simulink model "MATE_SynchronousMachine"  (R2024b)
settings: Solver=FixedStepDiscrete  StartTime=0.0  StopTime=6  FixedStep=Ts  RelTol=1e-4  EnableMultiTasking=on
PostLoadFcn:
  | Ts=25e-6;offset=4;
InitFcn:
  | Ts=25e-6;offset=4;
undefined symbols (not defined in the file): DiscIntNeverNeededParam, MATE, Phase, Rsnu, Single
libraries: fl_lib x58, nesl_utility x43, ee_lib x13, simetran x5, simetranss x3, powerlib_extras x3, simulink_extras x2, simulink x2
(part 1 of 4)
settings Model: ARTEMISmethode_block_infos=$$__separator__$$  Creator=by2815  LastModifiedBy=CD8435
settings SolverCC: AlgebraicLoopSolver=TrustRegion
settings DataIOCC: SaveFormat=Structure  SignalLoggingSaveFormat=ModelDataLogs  SaveOutput=off  SignalLogging=off  SaveTime=off  ReturnWorkspaceOutputs=off  SignalLoggingName=sigsOut
settings OptimizationCC: ExpressionDepthLimit=2147483647  InitFltsAndDblsToZero=on  LifeSpan=inf
settings DebuggingCC: SaveWithParameterizedLinksMsg=none  UnderspecifiedInitializationDetection=Classic  MergeDetectMultiDrivingBlocksExec=none  SignalResolutionControl=TryResolveAllWithWarning  MultiTaskDSMMsg=warning  MultiTaskCondExecSysMsg=none  FcnCallInpInsideContextMsg=warning  AllowSymbolicDim=off  StateNameClashWarn=warning  NonBusSignalsTreatedAsBus=error  SFUnexpectedBacktrackingDiag=warning  SFNoUnconditionalDefaultTransitionDiag=warning  SFExecutionAtInitializationDiag=none  ArithmeticOperatorsInVariantConditions=warning
settings HardwareCC: ProdBitPerPointer=32  ProdBitPerSizeT=32  ProdBitPerPtrDiffT=32  ProdLargestAtomicFloat=None  ProdIntDivRoundTo=Undefined  ProdEndianess=Unspecified  ProdWordSize=32  ProdHWDeviceType=32-bit Generic  TargetUnknown=on
settings ModelReferenceCC: EnableRefExpFcnMdlSchedulingChecks=on  PropagateSignalLabelsOutOfModel=off
settings SFSimCC: SimUseLocalCustomCode=off  CustomCodeUndefinedFunction=UseInterfaceOnly
settings RTWCC: RTWUseLocalCustomCode=off  GPUComputeCapability=3.5
settings CodeAppCC: StateflowObjectComments=on
settings GRTTargetCC: TargetFcnLib=ansi_tfl_tmw.mat  TargetLangStandard=C89/C90 (ANSI)  CombineOutputUpdateFcns=off  GRTInterface=on
settings ConfigComp: CovMetricSettings=dw  CovSaveCumulativeToWorkspaceVar=on  CovSaveSingleToWorkspaceVar=on  CovExternalEMLEnable=off
settings SimscapeCC: SimscapeNormalizeSystem=off

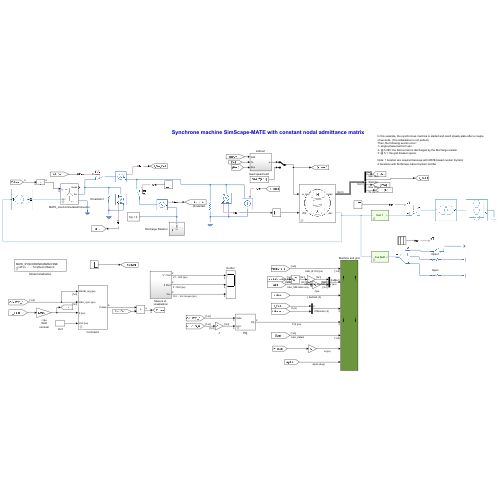
[thumbnail: Simulink's stored preview of the top-level diagram]
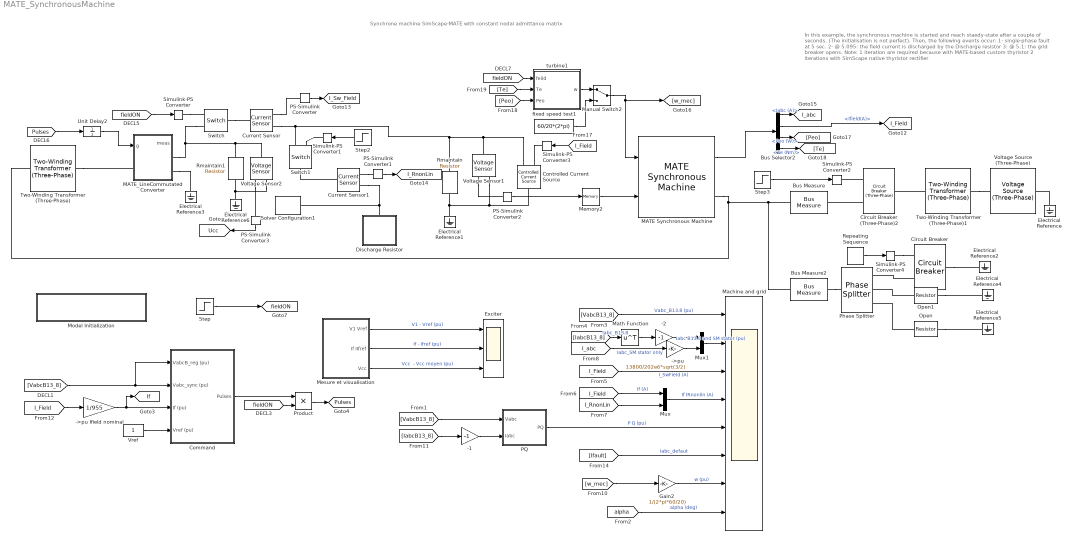
== system MATE_SynchronousMachine ==
  note: In this example, the synchronous machine is started and reach staedy-state after a couple of seconds. (The initialisation is not perfect).
      | Then, the following events occur:
      | 1- single-phase fault at 5 sec.
      | 2- @ 5.095: the field current is discharged by the Discharge resistor
      | 3: @ 5.1: the grid breaker opens.
      |
      | Note: 1 iteration are required because with MATE-based custom thyristor
      | 2 iterations with SimScape native thyristor rectifier
  note: Synchrone machine SimScape-MATE with constant nodal admittance matrix
  -1 : Gain  Gain=-1
  -2 : Gain  Gain=-1
  ->pu : Gain  Gain=13800/202e6*sqrt(3/2)
  ->pu Ifield nominal : Gain  Gain=1/955
  Bus Selector2 : BusSelector  OutputSignals=Iabc (A),Ifield(A),Peo (W),Te (Nm)
  Bus Measure : simetranss/Measure/Bus Measure  VoltageMeasurement=phase-to-ground  SetLabelV=on  LabelV=VabcB13_8  Vpu=on  VpuLL=off  CurrentMeasurement=yes  SetLabelI=on  LabelI=IabcB13_8  Ipu=on  Pbase=202e6  Vbase=13.8e3  bnumber=1  dis=off
  Bus Measure2 : simetranss/Measure/Bus Measure  VoltageMeasurement=phase-to-ground  SetLabelV=on  LabelV=Vfault  Vpu=off  VpuLL=off  CurrentMeasurement=yes  SetLabelI=on  LabelI=Ifault  Ipu=off  Pbase=202e6  Vbase=13.8e3  bnumber=fault  dis=off
  Circuit Breaker : ee_lib/Switches & Breakers/Circuit Breaker  R_closed=0.01 Ohm  G_open=1e-6 1/Ohm  threshold=0.5 V  breaker_behavior=ee.enum.switches.breakerBehavior.zeroCrossingEnable
      settings: InternalSimscapePortConfiguration="{\"Bottom\":[],\"Left\":[{\"id\":\"vT\",\"label\":\"vT\",\"type\":\"input\"},{\"id\":\"p1\",\"label\":\"\",\"type\":\"foundation.electrical.electrical\"}],\"Right\":[{\"id\":\"p2\",\"label\":\"\",\"type\":\"foundation.electrical.electrical\"}],\"Top\":[]}"
  Circuit Breaker (Three-Phase)2 : ee_lib/Switches & Breakers/Circuit Breaker (Three-Phase)  R_closed=0.01 Ohm  G_open=1e-6 1/Ohm  threshold=0.5 V  breaker_behavior=ee.enum.switches.breakerBehavior.zeroCrossingEnable
      settings: InternalSimscapePortConfiguration="{\"Bottom\":[],\"Left\":[{\"id\":\"vT\",\"label\":\"vT\",\"type\":\"input\"},{\"id\":\"N1\",\"label\":\"~1\",\"type\":\"foundation.electrical.three_phase\"}],\"Right\":[{\"id\":\"N2\",\"label\":\"~2\",\"type\":\"foundation.electrical.three_phase\"}],\"Top\":[]}"
  Command : Subsystem  mask{ModOp=Automatique (regulation de tension), Vref=1.0, Iref_man=1.0, K_V=[ 20 300  ], K_I=[ 400  1000 ], Ts=Ts}
      mask prompts: ModOp "Mode d'operation"; Vref "Consigne de tension (pu)"; Iref_man "Consigne de courant (pu)"; K_V "Gain du regulateur de tension [ Kp  Ki ]"; K_I "Gain du regulateur de courant: [ Kp  Ki ]"; Ts "Pas de calcul"
      mask init:
      | Kp_V=K_V(1); Ki_V=K_V(2);
      | Kp_I=K_I(1); Ki_I=K_I(2);
      | if ModOp==1
      |     Auto=1;
      | else
      |     Auto=0;
      | end
      mask TypeOptions ModOp: Automatique (regulation de tension) | Manuel (regulation de courant)
  Controlled Current Source : fl_lib/Electrical/Electrical Sources/Controlled Current Source
  Current Sensor : fl_lib/Electrical/Electrical Sensors/Current Sensor
  Current Sensor1 : fl_lib/Electrical/Electrical Sensors/Current Sensor
  Discharge Resistor : Subsystem
  Electrical Reference{,1..6} (7 alike) : fl_lib/Electrical/Electrical Elements/Electrical Reference
  Exciter : Scope  NumInputPorts=3
  Gain2 : Gain  Gain=1/(2*pi*60/20)
  MATE Synchronous Machine : simetranss/Machines/MATE Synchronous Machine  NominalParameters="[ 202e6  13800   60   955 ]"  Rtype=Salient (5ft order model)  Stator="[ 2.9069E-03  3.0892E-04  3.2164E-03 9.7153E-04 0.0]"  Field="[ 5.9013E-04*0.128/0.08381   3.0712E-04]"  Dampers1="[ 1.1900E-02  4.9076E-04   2.0081E-02  1.0365E-03  2.0081E-02  1.0365E-03]"  PolePairs=20  InitialConditions=-95  InitCurrents=[ 1180 9560 9560 9650 [0 -120 120]-95]  Ts=Ts  sat=on  DiffSat=off  SatVt=[0 0.7 1 1.4]  SatIfd=[0 0.5 1 2]  plotsat=off  R0=500  X0=0.11643  nsnf_readonly=0.083912
  MATE_LineCommutatedConverter : Subsystem  AncestorBlock=simetran/MATE_LineCommutatedConverter  mask(MATE 3-phase Diode/Thyristor Rectifier){umate=on, sd=Thyristors, ron=1e-2, roff=1e5, vf=1, rcs=on, rsnu=100, csnu=2e-6, ts=Ts}
      mask prompts: umate "Use MATE aggregated model"; sd "Switching Device"; ron "Ron (Ohms)"; roff "Roff (Ohms)"; vf "Forward voltage drop (V)"; rcs "RC snubber (otherwise only R)"; rsnu "Snubber resistance (Ohms)"; csnu "Snubber capacitance (Ohms)"; ts "Sample time (s)"
      mask init:
      | bloc=gcb;
      | 
      | if isequal(get_param(bloc,'rcs'), 'on')
      |     RCsnubber=1;
      | else
      |     RCsnubber=0;
      | end
      | bloc=gcb;
      | um=get_param(bloc,'umate');
      | if isequal (um,'on')
      | [MATE,MATERT]=Compute_6_pulse_thy_Fnc(bloc, 4, rsnu,csnu, RCsnubber,ron,ts,1,vf);
      | end
      mask Callback umate:
      | bloc=gcb;
      | um=get_param(bloc,'umate');
      | if isequal (um,'on')
      |     set_param([bloc '/MATE_AGGREG'], 'Commented', 'off');
      |     set_param([bloc '/MATEPREP'], 'Commented', 'on');
      | else
      |     set_param([bloc '/MATE_AGGREG'], 'Commented', 'on');
      |     set_param([bloc '/MATEPREP'], 'Commented', 'off');
      | end
      mask TypeOptions sd: Diodes | Thyristors
  Machine and grid : Scope  NumInputPorts=8
  Manual Switch2 : ManualSwitch
  Math Function : Math  Operator=transpose
  Memory2 : Memory
  Mesure et visualisation : Subsystem
  Model Initialization : Subsystem  AncestorBlock=artemis/Tools /Misc/Model Initialization  mask(Model Functions){InitFcnX=Ts=25e-6;offset=4;, prel=off, posl=on, inif=on, strf=off}
      mask prompts: InitFcnX "Initialisation"; prel "Preload Function"; posl "PostLoad Function"; inif "InitFcn"; strf "StartFcn"
      mask init:
      | currentBlock = gcb;
      | root = bdroot(currentBlock);
      | 
      | if ~strcmp(get_param(root,'BlockDiagramType'),'library')
      |     if prel==1
      |         set_param(root, 'PreLoadFcn', InitFcnX);
      |     else
      |         set_param(root, 'PreLoadFcn', '');
      |     end
      |     if inif==1
      |         set_param(root, 'InitFcn', InitFcnX);
      |     else
      |         set_param(root, 'InitFcn', '');
      |     end
      |     if strf==1
      |         set_param(root, 'StartFcn', InitFcnX);
      |     else
      |         set_param(root, 'StartFcn', '');
      |     end
      |     if posl==1
      |         set_param(root, 'PostLoadFcn', InitFcnX);
      |     else
      |         set_param(root, 'PostLoadFcn', '');
      |     end
      | end
      | 
      | pos = get_param(currentBlock, 'Position');
      | width = pos(3) - pos(1); height = pos(4) - pos(2);
      | txt = [ upper(root) '\n' '- InitFcn. . . . . '  get_param(root, 'InitFcn') ];
      settings: CopyFcn=set_param(gcb,'LinkStatus','inactive')
      mask Display: text(5, height*0.5, txt, 'horizontalAlignment', 'left', 'verticalAlignment', 'middle') ;
  Mux : Mux  Inputs=2
  Mux1 : Mux  Inputs=2
  Open : fl_lib/Electrical/Electrical Elements/Resistor  R=1e8 Ohm  i_specify=off  i_priority=None  i=0 A  i_nominal_specify=off  i_nominal_value=1  i_nominal_unit=A  v_specify=off  v_priority=None  v=0 V  v_nominal_specify=off  v_nominal_value=1  v_nominal_unit=V
  Open1 : fl_lib/Electrical/Electrical Elements/Resistor  R=1e8 Ohm  i_specify=off  i_priority=None  i=0 A  i_nominal_specify=off  i_nominal_value=1  i_nominal_unit=A  v_specify=off  v_priority=None  v=0 V  v_nominal_specify=off  v_nominal_value=1  v_nominal_unit=V
  PQ : Subsystem  mask(3-phase instantaneous active and reactive power){}
      mask init:
      | power_initmask();
      mask Display: disp('')
  PS-Simulink Converter{,1..3} (4 alike) : nesl_utility/PS-Simulink Converter  PhysicalDomain=network_engine_domain  SubClassName=ps_output  LeftPortType=input  RightPortType=output  PseudoPeriodic=off  Frequencies=[]  VectorFormat=inherit  Unit=inherit  AffineConversion=off
  Phase Splitter : ee_lib/Connectors & References/Phase Splitter
  Product : Product
  Repeating Sequence : simulink/Sources/Repeating Sequence  rep_seq_t="[0   [1-Ts 1  1.15-Ts 1.15]+offset  100]"  rep_seq_y="[1     1    0      0        1                1]"
  Rmaintain : fl_lib/Electrical/Electrical Elements/Resistor  R=5000 Ohm  i_specify=off  i_priority=None  i=0 A  i_nominal_specify=off  i_nominal_value=1  i_nominal_unit=A  v_specify=off  v_priority=None  v=0 V  v_nominal_specify=off  v_nominal_value=1  v_nominal_unit=V
  Rmaintain1 : fl_lib/Electrical/Electrical Elements/Resistor  R=50000 Ohm  i_specify=off  i_priority=None  i=0 A  i_nominal_specify=off  i_nominal_value=1  i_nominal_unit=A  v_specify=off  v_priority=None  v=0 V  v_nominal_specify=off  v_nominal_value=1  v_nominal_unit=V
  Simulink-PS Converter{,1..4} (5 alike) : nesl_utility/Simulink-PS Converter  PhysicalDomain=network_engine_domain  SubClassName=ps_input  LeftPortType=input  RightPortType=output  PseudoPeriodic=off  Frequencies=[]  NoiseDistribution=none  NoiseParameters=[]  Unit=1  AffineConversion=off  FilteringAndDerivatives=provide  SimscapeFilterOrder=1  InputFilterTimeConstant=0.001  UdotUserProvided=0
  Solver Configuration1 : nesl_utility/Solver Configuration  PhysicalDomain=network_engine_domain  SubClassName=solver  LeftPortType=input  RightPortType=generic  Tones=[]  Harmonics=[]  SimulateNoise=off  Profile=off  UseLocalSampling=off  EnableSwitchedLinearOptims=on  FrequencyDomain=off  UseCCode=off  RelTol=0.001  AbsTol=1e-06  MinStep=1e-09  ToWorkspace=off  RevertToSquareIcSolve=off  NumHomotopyIterations=100  PhasorMode=off  PhasorModeNumHarmonics=1  ConsistencySolver=NEWTON_FTOL  IndexReductionMethod=DerivativeReplacement  DoDC=off  ResidualTolerance=0.001  ConsistencyTolSource=GLOBAL  ConsistencyAbsTol=0.001  ConsistencyRelTol=0.001  ConsistencyTolFactor=0.001  UseLocalSolver=on  LocalSolverChoice=NE_BACKWARD_EULER_ADVANCER  ResolveIndetEquations=off  FunctionEvalNumThread=1  LocalSolverSampleTime=Ts  DoFixedCost=on  MaxNonlinIter=1  MaxModeIter=2  ComputeImpulses=off  ImpulseIterations=2  LinearAlgebra=Sparse  LinearAlgebraNumThread=0  EquationFormulation=NE_TIME_EF  DelaysMemoryBudget=1024  AutomaticFiltering=off  FilteringTimeConstant=0.001  PartitionStorageMethod=AS_NEEDED  PartitionMemoryBudget=1024  PartitionMethod=ROBUST  MultibodyUseLocalSolver=off  MultibodyLocalSolverChoice=ODE1  MultibodyLocalSolverSampleTime=0.001
  Step : Step  Time=1.1+offset  Before=1  After=0  SampleTime=0
  Step2 : Step  Time=1.095+offset  SampleTime=0
  Step3 : Step  Time="[ 1.1+offset  ]"  SampleTime=0
  Switch : fl_lib/Electrical/Electrical Elements/Switch  R_closed=0.01 Ohm  G_open=1e-8 1/Ohm  Threshold=0.5  i_specify=off  i_priority=None  i=0 A  i_nominal_specify=off  i_nominal_value=1  i_nominal_unit=A  v_specify=off  v_priority=None  v=0 V  v_nominal_specify=off  v_nominal_value=1  v_nominal_unit=V
  Switch1 : fl_lib/Electrical/Electrical Elements/Switch  R_closed=0.01 Ohm  G_open=1e-8 1/Ohm  Threshold=0.5  i_specify=off  i_priority=None  i=0 A  i_nominal_specify=off  i_nominal_value=1  i_nominal_unit=A  v_specify=off  v_priority=None  v=0 V  v_nominal_specify=off  v_nominal_value=1  v_nominal_unit=V
  Two-Winding Transformer (Three-Phase) : ee_lib/Passive/Transformers/Two-Winding Transformer (Three-Phase)  SRated=3.4e6 A*V  FRated=60 Hz  Winding1Connection=ee.enum.windingconnection.Yg  VRated1=13800 V  Winding2Connection=ee.enum.windingconnection.delta1  VRated2=1221 V  CoreType=ee.enum.coretype.fivelimb  pu_Rw1=0.001  pu_Rw2=0.001  leakage_reactance_option=ee.enum.transformer_leakage.include  pu_Xl1=0.03  pu_Xl2=0.03  magnetizing_resistance_option=ee.enum.transformer_magnetizingResistance.include  pu_Rm=500  magnetizing_reactance_option=ee.enum.transformer_magnetizingReactance.include  saturation_option=ee.enum.transformer_saturation.exclude  pu_Xm=500  current_data=[0, .002, 1, 2]  magnetic_flux_data=[0, 1.2, 1.5, 1.51]  pu_X0=0.5  i1_specify=on  i1_priority=High  i1=[0, 0, 0] A  i1_nominal_specify=off  i1_nominal_value=1  i1_nominal_unit=A  i2_specify=on  i2_priority=High  i2=[0, 0, 0] A  i2_nominal_specify=off  i2_nominal_value=1  i2_nominal_unit=A  phi_specify=off  phi_priority=None  phi=[0, 0, 0]  phi_nominal_specify=off  phi_nominal_value=1  phi_nominal_unit=1  power_dissipated_specify=off  power_dissipated_priority=None  power_dissipated=0 W  power_dissipated_nominal_specify=off  power_dissipated_nominal_value=1  power_dissipated_nominal_unit=W
      settings: InternalSimscapePortConfiguration="{\"Bottom\":[],\"Left\":[{\"id\":\"N1\",\"label\":\"~1\",\"type\":\"foundation.electrical.three_phase\"}],\"Right\":[{\"id\":\"N2\",\"label\":\"~2\",\"type\":\"foundation.electrical.three_phase\"}],\"Top\":[]}"
  Two-Winding Transformer (Three-Phase)1 : ee_lib/Passive/Transformers/Two-Winding Transformer (Three-Phase)  SRated=390e6 A*V  FRated=60 Hz  Winding1Connection=ee.enum.windingconnection.delta1  VRated1=13800 V  Winding2Connection=ee.enum.windingconnection.Yg  VRated2=735e3 V  CoreType=ee.enum.coretype.fivelimb  pu_Rw1=0.001  pu_Rw2=0.001  leakage_reactance_option=ee.enum.transformer_leakage.include  pu_Xl1=0.149  pu_Xl2=0.0001  magnetizing_resistance_option=ee.enum.transformer_magnetizingResistance.include  pu_Rm=500  magnetizing_reactance_option=ee.enum.transformer_magnetizingReactance.include  saturation_option=ee.enum.transformer_saturation.exclude  pu_Xm=500  current_data=[0, .002, 1, 2]  magnetic_flux_data=[0, 1.2, 1.5, 1.51]  pu_X0=0.5  i1_specify=on  i1_priority=High  i1=[0, 0, 0] A  i1_nominal_specify=off  i1_nominal_value=1  i1_nominal_unit=A  i2_specify=on  i2_priority=High  i2=[0, 0, 0] A  i2_nominal_specify=off  i2_nominal_value=1  i2_nominal_unit=A  phi_specify=off  phi_priority=None  phi=[0, 0, 0]  phi_nominal_specify=off  phi_nominal_value=1  phi_nominal_unit=1  power_dissipated_specify=off  power_dissipated_priority=None  power_dissipated=0 W  power_dissipated_nominal_specify=off  power_dissipated_nominal_value=1  power_dissipated_nominal_unit=W
      settings: InternalSimscapePortConfiguration="{\"Bottom\":[],\"Left\":[{\"id\":\"N1\",\"label\":\"~1\",\"type\":\"foundation.electrical.three_phase\"}],\"Right\":[{\"id\":\"N2\",\"label\":\"~2\",\"type\":\"foundation.electrical.three_phase\"}],\"Top\":[]}"
  Unit Delay2 : UnitDelay  InitialCondition=[1 0 0 1 0 0]  SampleTime=Ts  HasFrameUpgradeWarning=on
  Voltage Source (Three-Phase) : ee_lib/Sources/Voltage Source (Three-Phase)  vline_rms=735e3 V  shift=0 deg  freq=60 Hz  impedance_option=1  SShortCircuit=10000e6 A*V  XR=15  R=0.01 Ohm  L=3.97e-4 H  harmonic_option=0  harmonic_orders=[5, 7, 11, 13]  harmonic_ratios=[.1, .1, .1, .1]  G_parasitic=0 1/Ohm  I_specify=on  I_priority=High  I=[0, 0, 0] A  I_nominal_specify=off  I_nominal_value=1  I_nominal_unit=A
  Voltage Sensor1 : fl_lib/Electrical/Electrical Sensors/Voltage Sensor
  Voltage Sensor2 : fl_lib/Electrical/Electrical Sensors/Voltage Sensor
  Vref : Constant
  fixed speed test1 : Constant  Value=60/20*(2*pi)
  turbine1 : Subsystem
  tag scope: I_Field=global, I_RnonLin=global, I_Sw_Field=global, I_abc=global, If=global, Pulses=global, Ucc=global, fieldON=global
  wires:
  [VabcB13_8] -> Machine and grid/1  "Vabc_B13.8 (pu)"
  [IabcB13_8] -> Math Function/1  "Iabc_B13.8"
  [I_Field] -> Machine and grid/3  "I_SwField (A)"
  [I_Field] -> Mux/1  "If (A)"
  [I_RnonLin] -> Mux/2
  [w_mec] -> Gain2/1
  [Ifault] -> Machine and grid/6  "Iabc_defaut"
  [IabcB13_8] -> -1/1
  [VabcB13_8] -> PQ/1(Vabc)
  PQ/1(PQ) -> Machine and grid/5  "P Q (pu)"
  Vref/1 -> Command/4(Vref (pu))
  [alpha] -> Machine and grid/8  "alpha (deg)"
  Gain2/1 -> Machine and grid/7  "w (pu)"
  ->pu Ifield nominal/1 -> [If], Command/3(If (pu))
  -1/1 -> PQ/2(Iabc)
  Step/1 -> [fieldON]
  Command/1(Pulses) -> Product/1
  Product/1 -> [Pulses]
  [VabcB13_8] -> Command/1(VabcB_reg (pu)), Command/2(Vabc_sync (pu))
  [I_Field] -> ->pu Ifield nominal/1
  [fieldON] -> Product/2
  Mesure et visualisation/1(V1 Vref) -> Exciter/1  "V1 - Vref (pu)"
  Mesure et visualisation/2(If IIfref) -> Exciter/2  "If - Ifref (pu)"
  Mesure et visualisation/3(Vcc) -> Exciter/3  "Vcc  - Vcc moyen (pu)"
  -2/1 -> Mux1/1
  [I_abc] -> ->pu/1  "Iabc_SM stator only"
  Mux1/1 -> Machine and grid/2  "Iabc B13.8 and SM stator (pu)"
  Mux/1 -> Machine and grid/4  "If IRnonlin (A)"
  ->pu/1 -> Mux1/2
  [fieldON] -> Simulink-PS Converter/1
  Step2/1 -> Simulink-PS Converter1/1
  MATE Synchronous Machine/1 -> Bus Selector2/1
  Bus Selector2/2 -> [I_Field]  "<Ifield(A)>"
  Memory2/1 -> MATE Synchronous Machine/2
  PS-Simulink Converter2/1 -> Memory2/1
  Step3/1 -> Simulink-PS Converter2/1
  Bus Selector2/1 -> [I_abc]  "<Iabc (A)>"
  Bus Selector2/3 -> [Peo]  "<Peo (W)>"
  Bus Selector2/4 -> [Te]  "<Te (Nm)>"
  [Pulses] -> Unit Delay2/1
  PS-Simulink Converter/1 -> [I_Sw_Field]
  PS-Simulink Converter1/1 -> [I_RnonLin]
  [Te] -> turbine1/2(Te)
  [fieldON] -> turbine1/1(feild)
  Manual Switch2/1 -> MATE Synchronous Machine/1, [w_mec]
  fixed speed test1/1 -> Manual Switch2/2
  [Peo] -> turbine1/3(Peo)
  turbine1/1(w) -> Manual Switch2/1
  Math Function/1 -> -2/1
  PS-Simulink Converter3/1 -> [Ucc]
  [I_Field] -> Simulink-PS Converter3/1
  Unit Delay2/1 -> MATE_LineCommutatedConverter/1(g)
  Repeating Sequence/1 -> Simulink-PS Converter4/1
  connections:
  Switch/RConn2 -- MATE_LineCommutatedConverter/RConn1 -- Voltage Sensor2/LConn1 -- Rmaintain1/LConn1
  Simulink-PS Converter/RConn1 -- Switch/RConn1
  Switch/LConn1 -- Current Sensor/LConn1
  Simulink-PS Converter1/RConn1 -- Switch1/RConn1
  Rmaintain/LConn1 -- Current Sensor/RConn2 -- Switch1/RConn2 -- Controlled Current Source/RConn2 -- Voltage Sensor1/LConn1
  Current Sensor/RConn1 -- PS-Simulink Converter/LConn1
  Current Sensor1/LConn1 -- Switch1/LConn1
  Electrical Reference1/LConn1 -- Controlled Current Source/LConn1 -- Voltage Sensor1/RConn2 -- Rmaintain/RConn1
  Voltage Sensor1/RConn1 -- PS-Simulink Converter2/LConn1
  Simulink-PS Converter3/RConn1 -- Controlled Current Source/RConn1
  Two-Winding Transformer (Three-Phase)1/LConn1 -- Circuit Breaker (Three-Phase)2/RConn1
  Two-Winding Transformer (Three-Phase)1/RConn1 -- Voltage Source (Three-Phase)/RConn1
  Electrical Reference/LConn1 -- Voltage Source (Three-Phase)/LConn1
  Circuit Breaker (Three-Phase)2/LConn1 -- Simulink-PS Converter2/RConn1
  Simulink-PS Converter4/RConn1 -- Circuit Breaker/LConn1
  Current Sensor1/RConn1 -- PS-Simulink Converter1/LConn1
  MATE_LineCommutatedConverter/RConn2 -- Electrical Reference3/LConn1
  Open1/LConn1 -- Electrical Reference4/LConn1
  Open1/RConn1 -- Phase Splitter/RConn2
  Open/RConn1 -- Phase Splitter/RConn3
  Open/LConn1 -- Electrical Reference5/LConn1
  MATE Synchronous Machine/RConn1 -- Two-Winding Transformer (Three-Phase)/LConn1 -- Bus Measure2/RConn1 -- Bus Measure/RConn1
  Current Sensor1/RConn2 -- Solver Configuration1/RConn1 -- Discharge Resistor/LConn1
  Electrical Reference6/LConn1 -- Voltage Sensor2/RConn2 -- Rmaintain1/RConn1
  Voltage Sensor2/RConn1 -- PS-Simulink Converter3/LConn1
  Circuit Breaker/LConn2 -- Phase Splitter/RConn1
  Circuit Breaker/RConn1 -- Electrical Reference2/LConn1
  Two-Winding Transformer (Three-Phase)/RConn1 -- MATE_LineCommutatedConverter/LConn1
  Circuit Breaker (Three-Phase)2/LConn2 -- Bus Measure/LConn1
  Bus Measure2/LConn1 -- Phase Splitter/LConn1

== system MATE_SynchronousMachine/Command ==
  note: Excitation controller
  VabcB_reg (pu) : Inport
  Vabc_sync (pu) : Inport  Port=2
  If (pu) : Inport  Port=3
  Vref (pu) : Inport  Port=4
  Constant1 : Constant  Value=Iref_man
  Constant4 : Constant  Value=Auto
  Regulateur de courant : Subsystem
  Regulateur de tension (Mode automatique) : Subsystem
  Saturation : Saturate  UpperLimit=2.46  LowerLimit=0.33
  Switch : Switch  SaturateOnIntegerOverflow=off  InputSameDT=off
  "Synchro Generateur d'mpulsions " : Subsystem
  Pulses : Outport
  tag scope: Ifref=global, alpha=global
  wires:
  Vabc_sync (pu)/1 -> "Synchro Generateur d'mpulsions "/1(Vabc_138 (pu))
  "Synchro Generateur d'mpulsions "/1(P) -> Pulses/1
  VabcB_reg (pu)/1 -> Regulateur de tension (Mode automatique)/1(Vabc (pu))
  If (pu)/1 -> Regulateur de courant/1(If (pu))
  Constant4/1 -> Switch/2
  Constant1/1 -> Switch/3
  Regulateur de tension (Mode automatique)/1(Iref) -> Switch/1
  Switch/1 -> Saturation/1
  Saturation/1 -> [Ifref], Regulateur de courant/2(If_ref)
  Regulateur de courant/1(alpha) -> [alpha], "Synchro Generateur d'mpulsions "/2(alpha(deg))  "alpha (deg.)"
  Vref (pu)/1 -> Regulateur de tension (Mode automatique)/2(Vref)

== system MATE_SynchronousMachine/Discharge Resistor ==
  1-D Lookup Table : Lookup_n-D  NumberOfTableDimensions=1  BreakpointsForDimension1=[0 22 25 30 40 50 60 70 80 100 150 200 250 300 400 500 600 700 800 900 1000 1200]  Table="[0 22 25 30 40 50 60 70 80 100 150 200 250 300 400 500 600 700 800 900 1000 1200]./[1e-6 8.6250e-01 1.0500e+00 1.4250e+00 2.2500e+00 3.3750e+00 4.8750e+00 6.3750e+00 8.2500e+00  1.2000e+01 2.7750e+01 5.0250e+01 8.2500e+01 1.2000e+02 2.4000e+02 3.9750e+02 6.3750e+02 9.3750e+02 1.3125e+03 1.8000e+03 2.5500e+03 5.2500e+03]"  InternalRulePriority=Speed  RndMeth=Simplest
  Abs : Abs  SaturateOnIntegerOverflow=off
  Electrical Reference : fl_lib/Electrical/Electrical Elements/Electrical Reference
  Memory2 : Memory
  PS-Simulink Converter1 : nesl_utility/PS-Simulink Converter  PhysicalDomain=network_engine_domain  SubClassName=ps_output  LeftPortType=input  RightPortType=output  PseudoPeriodic=off  Frequencies=[]  VectorFormat=inherit  Unit=inherit  AffineConversion=off
  Simulink-PS Converter2 : nesl_utility/Simulink-PS Converter  PhysicalDomain=network_engine_domain  SubClassName=ps_input  LeftPortType=input  RightPortType=output  PseudoPeriodic=off  Frequencies=[]  NoiseDistribution=none  NoiseParameters=[]  Unit=1  AffineConversion=off  FilteringAndDerivatives=provide  SimscapeFilterOrder=1  InputFilterTimeConstant=0.001  UdotUserProvided=0
  Variable Resistor : fl_lib/Electrical/Electrical Elements/Variable Resistor  Rmin=0 Ohm  thermalEnable=false  thermal_mass=1 J/K  i_specify=off  i_priority=None  i=0 A  i_nominal_specify=off  i_nominal_value=1  i_nominal_unit=A  v_specify=off  v_priority=None  v=0 V  v_nominal_specify=off  v_nominal_value=1  v_nominal_unit=V  T_specify=off  T_priority=None  T=300 K  T_nominal_specify=off  T_nominal_value=1  T_nominal_unit=K
  Voltage Sensor : fl_lib/Electrical/Electrical Sensors/Voltage Sensor
  Conn1 : PMIOPort  Side=Left
  wires:
  PS-Simulink Converter1/1 -> Abs/1
  1-D Lookup Table/1 -> Memory2/1
  Memory2/1 -> Simulink-PS Converter2/1
  Abs/1 -> 1-D Lookup Table/1
  connections:
  Voltage Sensor/RConn2 -- Variable Resistor/RConn1 -- Electrical Reference/LConn1
  Voltage Sensor/RConn1 -- PS-Simulink Converter1/LConn1
  Voltage Sensor/LConn1 -- Conn1/RConn1 -- Variable Resistor/LConn2
  Simulink-PS Converter2/RConn1 -- Variable Resistor/LConn1

== system MATE_SynchronousMachine/MATE_LineCommutatedConverter ==
  g : Inport
  MATEPREP : Subsystem  Commented=on
  MATE_AGGREG : Subsystem
  Phase Splitter2 : ee_lib/Connectors & References/Phase Splitter
  abc : PMIOPort  Side=Left
  + : PMIOPort  Port=2  Side=Right
  - : PMIOPort  Port=3  Side=Right
  meas : Outport
  wires:
  g/1 -> MATEPREP/1(g), MATE_AGGREG/1(g)
  MATE_AGGREG/1(meas) -> meas/1
  connections:
  MATEPREP/RConn2 -- MATE_AGGREG/RConn2 -- -/RConn1
  MATEPREP/RConn1 -- MATE_AGGREG/RConn1 -- +/RConn1
  Phase Splitter2/RConn1 -- MATEPREP/LConn1 -- MATE_AGGREG/LConn1
  Phase Splitter2/RConn2 -- MATEPREP/LConn2 -- MATE_AGGREG/LConn2
  Phase Splitter2/RConn3 -- MATEPREP/LConn3 -- MATE_AGGREG/LConn3
  abc/RConn1 -- Phase Splitter2/LConn1

== system MATE_SynchronousMachine/Mesure et visualisation ==
  Discrete Mean value : Subsystem  mask(Discrete Mean value){Freq=60, Vinit=0, Ts=Ts}
      mask prompts: Freq "Fundamental frequency (Hz):"; Vinit "Initial input (DC component):"; Ts "Sample time:"
      mask help: Compute the mean value of the input signal over a running window of one cycle of the specified fundamental frequency.
      mask init:
      | SamplesPerCycle=1/Freq/Ts;
      | RoundSamplesPerCycle=ceil(SamplesPerCycle);
      | Delay=RoundSamplesPerCycle*Ts;
      | Corr1=(SamplesPerCycle-RoundSamplesPerCycle)/2;
      | Corr2=(SamplesPerCycle-RoundSamplesPerCycle)/SamplesPerCycle;
      | K1=Corr1*Corr2;
      | K2=Corr2 + Corr1*Corr2;
      mask Display: disp('Mean\n(discrete)')
  Mux : Mux  Inputs=2
  Mux3 : Mux  Inputs=2
  Mux4 : Mux  Inputs=2
  V1 Vref : Outport
  If IIfref : Outport  Port=2
  Vcc : Outport  Port=3
  wires:
  Discrete Mean value/1(Mean) -> Mux/2
  [Ucc] -> Mux/1, Discrete Mean value/1(In)
  Mux/1 -> Vcc/1  "Vcc - Vcc moyen (V)"
  [If] -> Mux3/1
  [Ifref] -> Mux3/2
  Mux3/1 -> If IIfref/1
  [V1] -> Mux4/1
  [Vref] -> Mux4/2
  Mux4/1 -> V1 Vref/1

== system MATE_SynchronousMachine/Model Initialization ==

== system MATE_SynchronousMachine/PQ ==
  note: 1) P = Va*Ia + Vb*Ib + Vc*Ic
  note: 2) Q = 1/sqrt(3)* (Vbc*Ia + Vca*Ib + Vab*Ic)
  note: This block computes the 3-phase instantaneous real power and reactive power using the following equations:
  note: Note: Equation 2 is valid only for a balanced and harmonic-free system.
  Vabc : Inport  PortDimensions=3
  Iabc : Inport  Port=2  PortDimensions=3
  Demux : Demux  Outputs=3
      settings: DisplayOption=none
  Mux : Mux  Inputs=3
  Mux1 : Mux  Inputs=2
  Product1 : Product  InputSameDT=on  SaturateOnIntegerOverflow=on  OutDataTypeStr=Inherit: Same as first input
  Product3 : Product  InputSameDT=on  SaturateOnIntegerOverflow=on  OutDataTypeStr=Inherit: Same as first input
  Sum : Sum  Inputs=+-  InputSameDT=on  SaturateOnIntegerOverflow=on  OutDataTypeStr=Inherit: Same as first input
  Sum1 : Sum  Inputs=1  InputSameDT=on  SaturateOnIntegerOverflow=on  OutDataTypeStr=Inherit: Same as first input
  Sum4 : Sum  Inputs=1  InputSameDT=on  SaturateOnIntegerOverflow=on  OutDataTypeStr=Inherit: Same as first input
  Sum5 : Sum  Inputs=+-  InputSameDT=on  SaturateOnIntegerOverflow=on  OutDataTypeStr=Inherit: Same as first input
  Sum6 : Sum  Inputs=+-  InputSameDT=on  SaturateOnIntegerOverflow=on  OutDataTypeStr=Inherit: Same as first input
  pu->V : Gain  Gain=1/sqrt(3)  SaturateOnIntegerOverflow=on  OutDataTypeStr=Inherit: Same as input  ParamDataTypeStr=Inherit: Same as input
  PQ : Outport  VectorParamsAs1DForOutWhenUnconnected=off
  wires:
  Sum1/1 -> pu->V/1
  Product3/1 -> Sum1/1
  Product1/1 -> Sum4/1
  Vabc/1 -> Product1/1, Demux/1
  Iabc/1 -> Product1/2, Product3/2
  Sum4/1 -> Mux1/1  "P"
  Demux/1 -> Sum/1, Sum6/2
  Demux/2 -> Sum/2, Sum5/1
  Demux/3 -> Sum5/2, Sum6/1
  Sum/1 -> Mux/3
  Sum5/1 -> Mux/1
  Sum6/1 -> Mux/2
  Mux/1 -> Product3/1
  pu->V/1 -> Mux1/2  "Q"
  Mux1/1 -> PQ/1

== system MATE_SynchronousMachine/turbine1 ==
  feild : Inport
  Te : Inport  Port=2
  Peo : Inport  Port=3
  Gain : Gain  Gain=1/(2*pi*60/20)
  Gain1 : Gain  Gain=1/202e6
  Gain3 : Gain  Gain=202e6
  Gain4 : Gain  Gain=1/(2*pi*60/20)
  Hydraulic Turbine and Governor : Subsystem  mask(Hydraulic Turbine and Governor){sm=[ 10/3  0.07 ], gate=[  0.01  0.97518  -0.1  0.1 ], reg=[  0.05  1.163  0.105  0  0.01  ], hyd=[  0  2.67  ], dref=0, po=0.802}
      mask prompts: sm "Servo-motor [ Ka()  Ta(sec) ]:"; gate "Gate opening limits [ gmin,gmax(pu)    vgmin,vgmax(pu/s) ]:"; reg "Permanent droop and regulator  [ Rp() Kp() Ki() Kd() Td(s) ]:"; hyd "Hydraulic turbine [ beta()  Tw(sec) ]:"; dref "Droop reference (0=power error, 1=gate opening):"; po "Initial mechanical power (pu):"
      mask help: Implements a hydraulic turbine combined to a PID governor system.
      mask init:
      | %block = gcb;
      | %[Ts, WantBlockChoice,ka,ta,gmin,gmax,vgmin,vgmax,Rp,Kp,ki,kd,td,beta,tw,go] = powericon('HydraulicTurbineInit',block,sm,gate,reg,hyd,po);
      | ka =sm (1 ); 
      | ta =sm (2 ); 
      | gmin =gate (1 ); 
      | gmax =gate (2 ); 
      | vgmin =gate (3 ); 
      | vgmax =gate (4 ); 
      | Rp =reg (1 ); 
      | kp =reg (2 ); 
      | ki =reg (3 ); 
      | kd =reg (4 ); 
      | td =reg (5 ); 
      | beta =hyd (1 ); 
      | tw =hyd (2 ); 
      | go =po *(gmax -gmin ); 
      | %powericon('SetInternalModels','set',block,WantBlockChoice);
      settings: OpenFcn=sps_rtmsupport('OpenFcn',gcbh)
      mask Help: helpview(psbhelp);
      mask Display: disp('')
  Mechanical model : Subsystem  mask(Synchronous machine mechanical model){J=3.4111e+06, F=0, fo=60/20, Ts=Ts}
      mask prompts: J "Inertia (kg.m^2)"; F "Friction (N.n.s)"; fo "Initial mechanical frequency (Hz)"; Ts "Sample Time (s)"
      mask help:
      | This is the mechanical equation of a synchronous machine.
      |
      | all values in SI.
      | J: inertia
      | F:friction
      | Te: torque input from the SM
      | Pin: power from the turbine
      | wmec: mechanical speed of the SM.
      | delta_wm: speed deviation
  Pref : Constant  Value=0.8
  Product1 : Product
  Terminator : Terminator
  wref : Constant
  w : Outport
  wires:
  Hydraulic Turbine and Governor/2(gate) -> Terminator/1
  Hydraulic Turbine and Governor/1(Pm) -> Gain3/1
  Gain1/1 -> Hydraulic Turbine and Governor/4(Pe0)
  Gain/1 -> Hydraulic Turbine and Governor/3(we)
  wref/1 -> Hydraulic Turbine and Governor/1(wref)
  Mechanical model/2(delta_wm) -> Gain4/1
  Pref/1 -> Product1/2
  Product1/1 -> Hydraulic Turbine and Governor/2(Pref)
  Gain3/1 -> Mechanical model/2(Pin)
  Mechanical model/1(wmec) -> Gain/1, w/1
  Gain4/1 -> Hydraulic Turbine and Governor/5(dw)
  feild/1 -> Product1/1
  Te/1 -> Mechanical model/1(Te)
  Peo/1 -> Gain1/1

== system MATE_SynchronousMachine/Command/Regulateur de courant ==
  If (pu) : Inport
  If_ref : Inport  Port=2
  Discrete 1st-Order Filter : Subsystem  mask(Discrete 1st-Order Filter){FilterType=Lowpass, Tc=1e-3, Ts=Ts, Initialize=off, Vac_Init=[0, 0, 60], Vdc_Init=0, PlotResponse=off, param1=[1 500 0.1]}
      mask prompts: FilterType "Filter Type:"; Tc "Time constant (s):"; Ts "Sample time:"; Initialize "Initialize filter states"; Vac_Init "AC initial input: [ Mag  Phase(degrees)  Freq(Hz) ]"; Vdc_Init "DC Initial input:"; PlotResponse "Plot filter response"; param1 "Frequency range(Hz) : [Start  End  Inc.]"
      mask init:
      | switch FilterType
      | case 1, % Lowpass
      |     X=[0 1 2 3 4];
      |     Y=[-2 -2 -3 -4 -4];
      |     numc=1;
      |     denc=[Tc 1];
      | case 2,   % Highpass
      |     X=[0 1 2 3 4];
      |     Y=[-4 -4 -3 -2 -2];
      |     numc=[1 0];
      |     denc=[1 1/Tc];
      | end
      | %
      | [Ac,Bc,Cc,Dc]=tf2ss(numc,denc);
      | %
      | %  Conversion to discrete transfer function
      | nstates = size(Ac,1);
      | if Ts<=0
      |     message = 'The Sample time parameter must be greater than zero. Note that specifying inherited sample time (-1) does not work for this block';
      |     error(message);
      | end
      | invexp = inv(eye(nstates) - (Ts/2)*Ac);
      | Ad = invexp*(eye(nstates) + (Ts/2)*Ac);
      | Bd = invexp*Bc;
      | Cd = Cc*invexp*Ts;
      | Dd = Cc*invexp*Bc*(Ts/2) + Dc;
      | %
      | if Initialize==1  % Compute initial conditions on states
      |     u1=Vac_Init(1)*exp(j*Vac_Init(2)*pi/180);
      |     u2=Vdc_Init*exp(j*90*pi/180);
      |     u=u1+u2;
      |     u0=imag(u); % input at  t=0;
      |     I=eye(size(Ac));
      |     sI1=I*j*(2*pi*Vac_Init(3));
      |     sI2=I*j*0;
      |     x=inv(sI1-Ac)*Bc*u1 + inv(sI2-Ac)*Bc*u2;
      |     x0c=imag(x);
      |     x0d=(I-Ac*Ts/2)*x0c/Ts - Bc/2*u0;
      | else
      |     x0d=0;
      | end
      | 
      | %
      | if PlotResponse==1 % Plot frequency and step response
      | t=[0:Tc/1000:7*Tc];
      | f=param1(1):param1(3):param1(2);
      | w=2*pi*f;
      | switch FilterType
      | 	case 1, % Lowpass
      | 		Ystep=1 - exp(-t/Tc);
      | 		RepFreq=1./(1+Tc*j.*w);
      | 	case 2,   % Highpass
      | 		Ystep=exp(-t/Tc);
      | 		RepFreq=1./(1 + (1./(Tc*j.*w)));
      | end
      | %
      | Mag=abs(RepFreq);
      | Pha=angle(RepFreq)*180/pi;
      | %
      | figure(1)
      | subplot(2,1,1)
      | plot(f,Mag)
      | grid
      | title('Bode Diagram')
      | ylabel('Magnitude')
      | subplot(2,1,2)
      | plot(f,Pha)
      | ylabel('Phase (deg)')
      | xlabel('Frequency (Hz)')
      | grid
      | figure(2)
      | plot(t,Ystep)
      | grid
      | ylabel('Amplitude')
      | xlabel('Time (s)')
      | title('Step Response')
      | end
      mask TypeOptions FilterType: Lowpass | Highpass
      mask Display: plot(X,Y);
  Discrete PI Controller1 : Subsystem  mask(Discrete PI Controller){Kp=400, Ki=1000, Par_Limits=[150 10], Init=79, Ts=Ts}
      mask prompts: Kp "Proportional gain (Kp):"; Ki "Integral gain (Ki):"; Par_Limits "Output limits: [ Upper   Lower ]"; Init "Output initial value:"; Ts "Sample time:"
      mask help: This block implements a basic discrete PI controller.
      mask init:
      | UpperLimit=Par_Limits(1);
      | LowerLimit=Par_Limits(2);
      mask Display: disp('PI');
  Sum : Sum  Inputs=|+-
  alpha : Outport
  wires:
  Discrete 1st-Order Filter/1(Out) -> Sum/1
  If (pu)/1 -> Discrete 1st-Order Filter/1(In)
  If_ref/1 -> Sum/2
  Sum/1 -> Discrete PI Controller1/1(Error)
  Discrete PI Controller1/1(Out) -> alpha/1

== system MATE_SynchronousMachine/Command/Regulateur de tension (Mode automatique) ==
  note: Regulateur de tension
  Vabc (pu) : Inport
  Vref : Inport  Port=2
  Discrete PI Controller1 : Subsystem  mask(Discrete PI Controller){Kp=Kp_V, Ki=Ki_V, Par_Limits=[2.46 0.33], Init=1, Ts=Ts}
      mask prompts: Kp "Proportional gain (Kp):"; Ki "Integral gain (Ki):"; Par_Limits "Output limits: [ Upper   Lower ]"; Init "Output initial value:"; Ts "Sample time:"
      mask help: This block implements a basic discrete PI controller.
      mask init:
      | UpperLimit=Par_Limits(1);
      | LowerLimit=Par_Limits(2);
      mask Display: disp('PI');
  Discrete 3-phase Positive-Sequence Fundamental Value : Subsystem  mask(Discrete 3-phase Positive-sequence fundamental value){Freq=60, Par_Init=[0 0], Ts=Ts}
      mask prompts: Freq "Fundamental frequency (Hz):"; Par_Init "Initial input (positive component): [ Mag  Phase(degrees) ]"; Ts "Sample time:"
      mask help: Compute the positive-sequence component of the input signal at the given fundamental frequency. The input is set of three balanced or unbalanced signals which may contain harmonics.
      mask init:
      | SamplesPerCycle=1/Freq/Ts;
      | RoundSamplesPerCycle=round(SamplesPerCycle);
      | Delay=RoundSamplesPerCycle*Ts - Ts/2;
      | Correction=SamplesPerCycle/RoundSamplesPerCycle - 1;
      | Real_Init=Par_Init(1)*cos(pi/180*Par_Init(2));
      | Imag_Init=Par_Init(1)*sin(pi/180*Par_Init(2));
      mask Display: disp('')
  Sum : Sum  Inputs=|-+
  Terminator : Terminator
  Iref : Outport
  tag scope: V1=global, Vref=global
  wires:
  Discrete 3-phase Positive-Sequence Fundamental Value/2(Phase) -> Terminator/1
  Vabc (pu)/1 -> Discrete 3-phase Positive-Sequence Fundamental Value/1(abc)
  Discrete PI Controller1/1(Out) -> Iref/1
  Sum/1 -> Discrete PI Controller1/1(Error)
  Vref/1 -> Sum/2, [Vref]
  Discrete 3-phase Positive-Sequence Fundamental Value/1(Mag) -> Sum/1, [V1]

== system MATE_SynchronousMachine/Command/Synchro Generateur d'mpulsions  ==
  Vabc_138 (pu) : Inport
  alpha(deg) : Inport  Port=2
  Demux : Demux  Outputs=3
  Discrete 3-phase PLL : Subsystem  mask(Discrete 3-phase PLL){Fmin=45, Par_Init=[0 60], ParK=[ 180 3200 1 ], Ts=Ts, AGC=on}
      mask prompts: Fmin "Minimum frequency (Hz):"; Par_Init "Initial inputs:[ Phase(degrees)   Frequency(Hz) ]"; ParK "Regulator gains [ Kp  Ki  Kd ]"; Ts "Sample time:"; AGC "Enable Automatic Gain Control"
      mask help:
      | This Phase Locked Loop (PLL) system can be used  to synchronize on a set of variable frequency, three-phase sinusoidal signals. If the Automatic Gain Control is enabled, the input (phase error) of the PLL regulator is scaled according to the input signals magnitude.
      |
      | For optimal performance, the following settings are recommended:
      |   [ Kp Ki  Kd ] = [ 180  3200  1 ]
      |   "Enable Automatic Gain Control" checked
      |
      | Input 1: Vector containing the normalized three-phase signals [Va Vb Vc]
      | Output 1:  Measured frequency (Hz) = w/(2pi)
      | Output 2:  Ramp w.t varying between  0 and 2*pi,
      |      synchronized on zero crossings of the fundamental (positive-sequence) of phase A.
      | Output 3: Vector [sin(wt) cos(wt)]
      mask init:
      | Kp=ParK(1);
      | Ki=ParK(2);
      | if length(ParK)==2
      |     Kd=0;
      | else
      |     Kd=ParK(3);
      | end    
      | Phase_Init=Par_Init(1);
      | Finit=Par_Init(2);
      settings: OpenFcn=power_openblockproxy();
      mask Display: disp('')
  Discrete Synchronized 12-Pulse Generator : Subsystem  mask(Discrete synchronized 12-pulse generator){Delta=D1 (lagging), pwidth=20, Double_Pulse=on, Ts=Ts}
      mask prompts: Delta "Delta winding connection"; pwidth "Pulse width (degrees)"; Double_Pulse "Double pulsing"; Ts "Sample time"
      mask help:
      | Use this block to fire the 12 thyristors of a 12-pulse converter.
      | Outputs 1 and 2 are two vectors of 6 pulses (0-1) to be sent to the two 6-pulse half bridges connected respectively to the Wye(Y) and Delta (D1 or D11) connected windings of the YYD converter transformer.
      | Pulses are individually synchronized on the 6 commutation voltages and generated alpha degrees after the increasing zero-crossings of the commutation voltages. The D pulses are either lagging or leading the Y pulses by 30 degrees.
      |
      | Input 'alpha_deg' :  Alpha firing signal (degrees).
      | Inputs 'A,B,C' : Phase-to-ground synchronization voltages  measured at the  primary side of the converter transformer.
      | Input 'Freq' : Frequency of the synchronization voltages (use a constant or the Freq PLL output)
      | Input 'Block' allows  blocking of the pulses when the applied signal is non zero.
      |
      | When the 'Douple pulsing' option is checked, two pulses are sent to each thyristor: a 1st pulse when the alpha angle is reached, then a 2nd pulse 60 degrees later, when the next thyristor is fired.
      mask init:
      | if (Delta == 1)
      |     D1 = 1;
      | else
      |     D1 = 0;
      | end
      mask TypeOptions Delta: D1 (lagging) | D11 (leading)
      mask Display: plot(0,0,100,100,[80 62 62 47 47 30],[40 40 60 60 40 40]-5)
  Ground2 : Ground
  Terminator : Terminator
  Terminator1 : Terminator
  Terminator2 : Terminator
  P : Outport
  wires:
  Vabc_138 (pu)/1 -> Discrete 3-phase PLL/1(Vabc(pu)), Demux/1
  Ground2/1 -> Discrete Synchronized 12-Pulse Generator/6(Block)
  alpha(deg)/1 -> Discrete Synchronized 12-Pulse Generator/1(alpha_deg)
  Demux/1 -> Discrete Synchronized 12-Pulse Generator/2(A)
  Demux/2 -> Discrete Synchronized 12-Pulse Generator/3(B)
  Demux/3 -> Discrete Synchronized 12-Pulse Generator/4(C)
  Discrete 3-phase PLL/1(Freq) -> Discrete Synchronized 12-Pulse Generator/5(Freq)
  Discrete Synchronized 12-Pulse Generator/2(PD) -> P/1
  Discrete 3-phase PLL/2(wt) -> Terminator/1
  Discrete 3-phase PLL/3(Sin_Cos) -> Terminator1/1
  Discrete Synchronized 12-Pulse Generator/1(PY) -> Terminator2/1

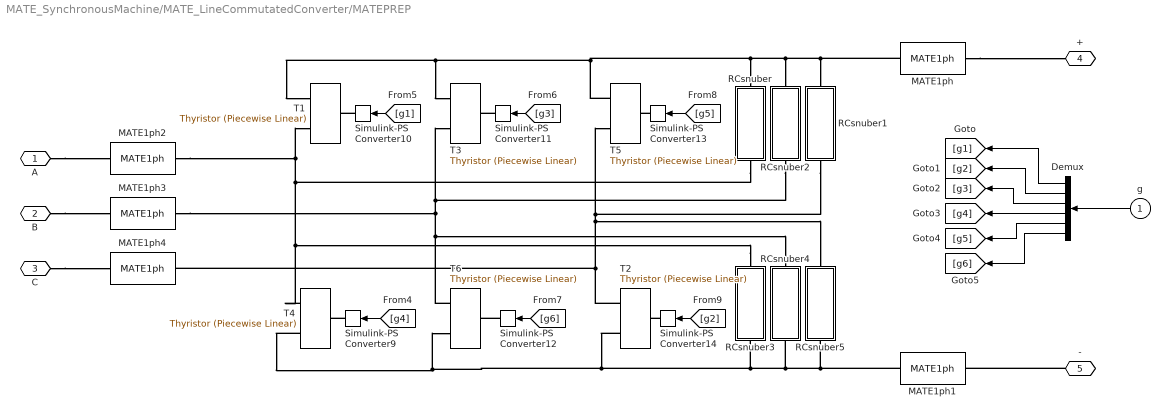
== system MATE_SynchronousMachine/MATE_LineCommutatedConverter/MATEPREP ==
  g : Inport
  Demux : Demux  Outputs=6
  MATE1ph : simetran/MATE1ph  bn=4  conty=Single-Phase  it=auto  Rse=1e-4  Rsh=1e9
      settings: AttributesFormatString=# %<bn>
  MATE1ph1 : simetran/MATE1ph  bn=5  conty=Single-Phase  it=auto  Rse=1e-4  Rsh=1e9
      settings: AttributesFormatString=# %<bn>
  MATE1ph2 : simetran/MATE1ph  bn=1  conty=Single-Phase  it=auto  Rse=1e-4  Rsh=1e9
      settings: AttributesFormatString=# %<bn>
  MATE1ph3 : simetran/MATE1ph  bn=2  conty=Single-Phase  it=auto  Rse=1e-4  Rsh=1e9
      settings: AttributesFormatString=# %<bn>
  MATE1ph4 : simetran/MATE1ph  bn=3  conty=Single-Phase  it=auto  Rse=1e-4  Rsh=1e9
      settings: AttributesFormatString=# %<bn>
  RCsnuber : Subsystem
  RCsnuber1 : Subsystem
  RCsnuber2 : Subsystem
  RCsnuber3 : Subsystem
  RCsnuber4 : Subsystem
  RCsnuber5 : Subsystem
  Simulink-PS Converter{9..14} (6 alike) : nesl_utility/Simulink-PS Converter  PhysicalDomain=network_engine_domain  SubClassName=ps_input  LeftPortType=input  RightPortType=output  PseudoPeriodic=off  Frequencies=[]  NoiseDistribution=none  NoiseParameters=[]  Unit=1  AffineConversion=off  FilteringAndDerivatives=provide  SimscapeFilterOrder=1  InputFilterTimeConstant=0.001  UdotUserProvided=0
  T{1..6} (6 alike) : ee_lib/Semiconductors & Converters/Thyristor (Piecewise Linear)  port_option=ee.enum.controlport.ps  Vf=0.8 V  Ron=0.001 Ohm  Goff=1e-5 1/Ohm  Vgt=0.5 V  Ih=1 A  diode_param=ee.enum.semiconductors.protectionDiode.external  diode_Vf=0.8 V  diode_Ron=0.001 Ohm  diode_Goff=1e-5 1/Ohm  diode_C=50e-9 F  diode_iRM=-235 A  diode_iF=300 A  diode_idot=-50 A/us  diode_trr_param=ee.enum.converters.diodetrr.trr_factor  diode_trr_factor=3  diode_trr=15 us  diode_Qrr=1500 s*uA  iak_specify=off  iak_priority=None  iak=0 A  iak_nominal_specify=off  iak_nominal_value=1  iak_nominal_unit=A  vak_specify=off  vak_priority=None  vak=0 V  vak_nominal_specify=off  vak_nominal_value=1  vak_nominal_unit=V  vgk_specify=off  vgk_priority=None  vgk=0 V  vgk_nominal_specify=off  vgk_nominal_value=1  vgk_nominal_unit=V  thermal_loss_option=ee.enum.converters.thermalLossOption.constantvalues  Von_data=[0, .1, .6, .8, 1, 1.3, 1.6, 2, 2.4; 0, .1, .7, 1, 1.2, 1.5, 1.9, 2.4, 2.8] V  Tj=[298.15, 398.15] K  Iout_data=[0, .1, 1, 5, 10, 20, 40, 70, 100] A  Eon_data=[0, .0024, .024, .12, .2, .48, 1.04, 2.16, 3.24; 0, .003, .03, .15, .25, .6, 1.3, 2.7, 4.05] * 1e-3 J  Tj_loss=[298.15, 398.15] K  Iout_data_loss=[0, .1, 1, 5, 10, 20, 40, 70, 100] A  Eon_scalar=22.86e-3 J  Eoff_natural_commutation=10e-3 J  Voff=300 V  Iout_scalar=600 A  onCurrentMeasDelay=1e-4 s  diodeModelType=ee.enum.converters.diodeModelType.pwl  diodeTableType=ee.enum.diode.tableType.IfMat  diode_IfMat=[.07, .12, .19, 1.75, 4.24, 7.32, 11.2; .16, .3, .72, 2.14, 4.02, 6.35, 9.12] A  diode_VfMat=[.9, 1.15, 1.25, 1.5, 1.75, 2.17, 2.6, 2.85; .58, .68, .75, 1.1, 1.38, 1.77, 2.27, 2.7] V  diode_TjVec=[25, 125] degC  diode_VfVec=[.5, .7, .9, 1.3, 1.7, 2.1, 2.5] V  diode_IfVec=[.1, .2, .5, 1, 2, 4, 7, 10] A  diode_rec_loss_model=ee.enum.diode.reverseRecoveryModel.fixed  diode_ErecVal=0 J  diode_scaleWithIandV=true  diode_ErecMat=zeros(2, 3) J  diode_TjrecVec=[298.15, 398.15] K  diode_IfrecVec=[.1, 1, 10] A  diode_IrecVal=10 A  diode_VrecVal=10 V  diode_tFilter=1 / 1000 / 100 s  thermal_network_parameterization=ee.enum.thermalNetworkTopology.external  Rth=[.08, .5] K/W  Rth_Cauer=[.08, .1, .5] K/W  Rth_Foster=[.08, .14, .22, .16] K/W  thermal_mass_parameterization=ee.enum.thermalNetwork.timeconstant  thermal_mass=[.01, .5] J/K  thermal_mass_Cauer=[.01, .1, .5] J/K  thermal_mass_Foster=[.001, .005, .05, .5] J/K  thermal_time_constant=[.001, .2] s  thermal_time_constant_Cauer=[.001, .1, .2] s  thermal_time_constant_Foster=[7e-05, .0007, .01, .08] s  thermal_mass_initial_temperatures=[25, 25] degC  thermal_mass_initial_temperatures_Cauer=[25, 25, 25] degC  junction_thermal_mass=0.01 J/K  Tvec_initial_Foster=[25, 25, 25, 25] degC  junction_temperature_specify=off  junction_temperature_priority=None  junction_temperature=25 degC  junction_temperature_nominal_specify=off  junction_temperature_nominal_value=1  junction_temperature_nominal_unit=degC  Qj_specify=off  Qj_priority=None  Qj=0 W  Qj_nominal_specify=off  Qj_nominal_value=1  Qj_nominal_unit=W  accumulatedSwitchingLosses_specify=off  accumulatedSwitchingLosses_priority=None  accumulatedSwitchingLosses=0 J
      settings: InternalSimscapePortConfiguration="{\"Bottom\":[],\"Left\":[{\"id\":\"G\",\"label\":\"\",\"type\":\"input\"}],\"Right\":[{\"id\":\"A\",\"label\":\"\",\"type\":\"foundation.electrical.electrical\"},{\"id\":\"K\",\"label\":\"\",\"type\":\"foundation.electrical.electrical\"}],\"Top\":[]}"
  A : PMIOPort  Side=Left
  B : PMIOPort  Port=2  Side=Left
  C : PMIOPort  Port=3  Side=Left
  + : PMIOPort  Port=4  Side=Right
  - : PMIOPort  Port=5  Side=Right
  wires:
  Demux/5 -> [g5]
  Demux/6 -> [g6]
  Demux/4 -> [g4]
  Demux/3 -> [g3]
  Demux/2 -> [g2]
  Demux/1 -> [g1]
  g/1 -> Demux/1
  [g4] -> Simulink-PS Converter9/1
  [g1] -> Simulink-PS Converter10/1
  [g3] -> Simulink-PS Converter11/1
  [g6] -> Simulink-PS Converter12/1
  [g5] -> Simulink-PS Converter13/1
  [g2] -> Simulink-PS Converter14/1
  connections:
  RCsnuber3/LConn1 -- T4/RConn2 -- RCsnuber/RConn1 -- MATE1ph2/RConn1 -- T1/RConn1
  MATE1ph3/RConn1 -- RCsnuber2/RConn1 -- T3/RConn1 -- T6/RConn2 -- RCsnuber4/LConn1
  RCsnuber1/RConn1 -- T5/RConn1 -- T2/RConn2 -- MATE1ph4/RConn1 -- RCsnuber5/LConn1
  RCsnuber4/RConn1 -- MATE1ph1/RConn1 -- RCsnuber5/RConn1 -- T2/RConn1 -- T6/RConn1 -- T4/RConn1 -- RCsnuber3/RConn1
  MATE1ph/RConn1 -- T1/RConn2 -- T3/RConn2 -- T5/RConn2 -- RCsnuber/LConn1 -- RCsnuber2/LConn1 -- RCsnuber1/LConn1
  -/RConn1 -- MATE1ph1/LConn1
  A/RConn1 -- MATE1ph2/LConn1
  B/RConn1 -- MATE1ph3/LConn1
  C/RConn1 -- MATE1ph4/LConn1
  Simulink-PS Converter9/RConn1 -- T4/LConn1
  Simulink-PS Converter10/RConn1 -- T1/LConn1
  Simulink-PS Converter11/RConn1 -- T3/LConn1
  Simulink-PS Converter12/RConn1 -- T6/LConn1
  Simulink-PS Converter13/RConn1 -- T5/LConn1
  Simulink-PS Converter14/RConn1 -- T2/LConn1
  MATE1ph/LConn1 -- +/RConn1
